simulink model "encoder_test"  (R2018b)
settings: Solver=FixedStepDiscrete  StartTime=0.0  StopTime=inf  RelTol=1e-3
libraries: simulink x1
settings Model: Creator=hiterd  LastModifiedBy=hiterd

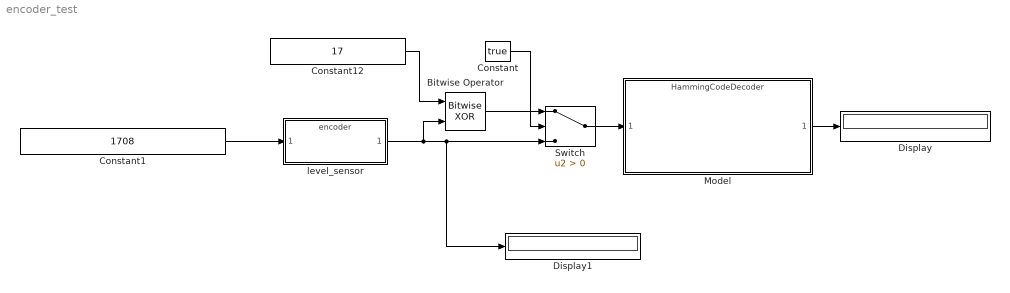
== system encoder_test ==
  Bitwise Operator : simulink/Logic and Bit Operations/Bitwise Operator  logicop=XOR  UseBitMask=off  NumInputPorts=2  BitMask=bin2dec('11011001')  BitMaskRealWorld=Stored Integer
  Constant : Constant  Value=true  SampleTime=-1
  Constant1 : Constant  Value=1708  OutDataTypeStr=int32  SampleTime=1
  Constant12 : Constant  Value=17  OutDataTypeStr=uint16  SampleTime=1
  Display : Display
  Display1 : Display
      settings: Format=binary (Stored Integer)
  Model : ModelReference  ModelNameDialog=HammingCodeDecoder.slx  SimulationMode=Normal  ModelReferenceVersion=1.4
  Switch : Switch  Criteria=u2 > Threshold
  level_sensor : ModelReference  ModelNameDialog=encoder.slx  SimulationMode=Normal  ModelReferenceVersion=1.48
  wires:
  Constant12/1 -> Bitwise Operator/1
  Bitwise Operator/1 -> Switch/1
  Switch/1 -> Model/1
  Constant/1 -> Switch/2
  Constant1/1 -> level_sensor/1
  Model/1 -> Display/1
  level_sensor/1 -> Bitwise Operator/2, Display1/1, Switch/3
